simulink model "WaterworldExample"  (R2016b)
settings: Solver=FixedStepAuto  StartTime=0.0  StopTime=100.0  FixedStep=0.01  RelTol=1e-3
settings Model: Creator=Thomas  LastModifiedBy=Thomas

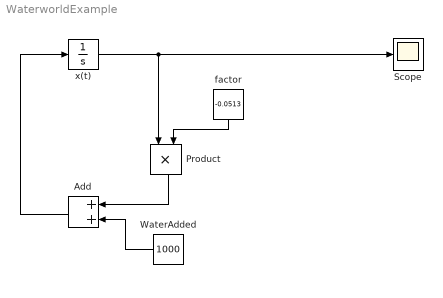
== system WaterworldExample ==
  Add : Sum
  Product : Product
  Scope : Scope
  WaterAdded : Constant  Value=1000
  factor : Constant  Value=-0.0513
  x(t) : Integrator  InitialCondition=100000
  wires:
  factor/1 -> Product/2
  x(t)/1 -> Scope/1, Product/1
  WaterAdded/1 -> Add/2
  Product/1 -> Add/1
  Add/1 -> x(t)/1
